simulink model "controlSpatialOrientation"  (R2025b)
settings: Solver=VariableStepAuto  StartTime=0.0  StopTime=100  RelTol=1e-3
undefined symbols (not defined in the file): C_T_pitch, C_T_rol, C_T_yaw, Ix, Iy, Iz
libraries: fuzblock x3
settings Model: Creator=torcik  LastModifiedBy=torcik

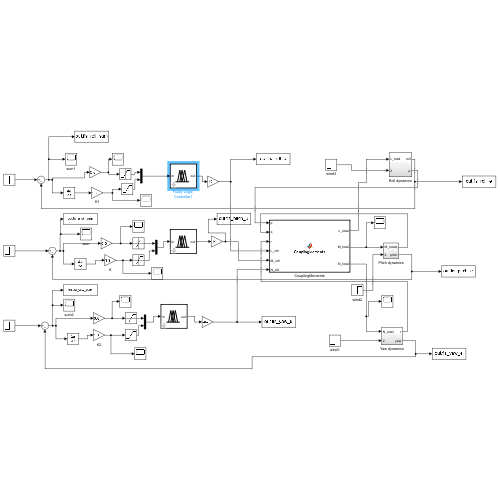
[thumbnail: Simulink's stored preview of the top-level diagram]
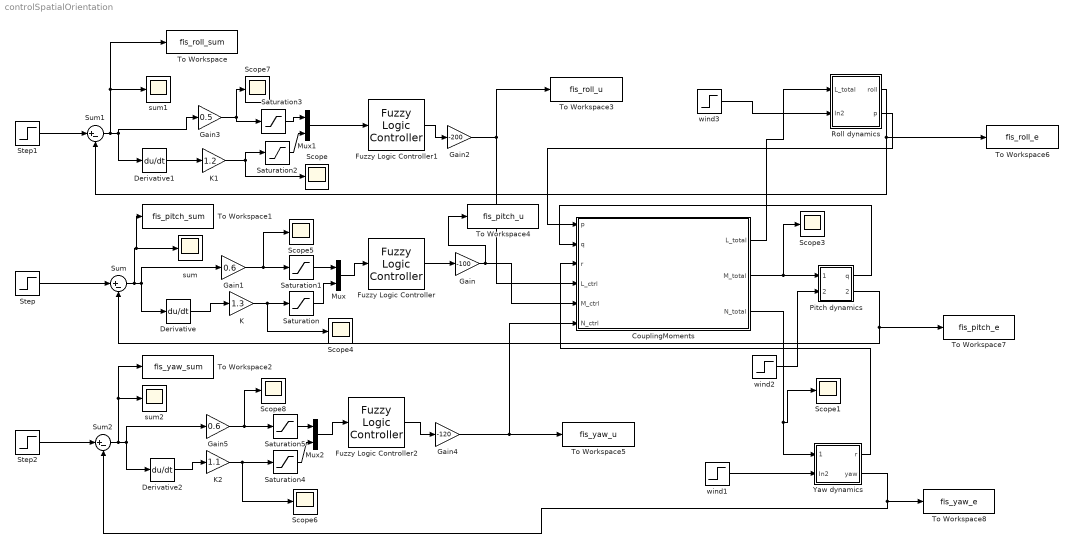
== system controlSpatialOrientation ==
  CouplingMoments : MATLAB Function  TreatAsAtomicUnit=on
  Derivative : Derivative
  Derivative1 : Derivative
  Derivative2 : Derivative
  Fuzzy Logic Controller : fuzblock/Fuzzy Logic  Controller  FIS='Mamdani_gauss'  OutputSampleNumber=101  DataType=double  UseLookupTable=off  NumBreakpoints=10  FuzzifiedInputs=off  RuleFiringStrengths=off  RuleOutputs=off  AggregatedOutputs=off  SimulateUsing=Interpreted execution  OutOfRangeInputValueMessage=warning  NoRuleFiredMessage=warning  EmptyOutputFuzzySetMessage=warning
  Fuzzy Logic Controller1 : fuzblock/Fuzzy Logic  Controller  FIS='Mamdani_gauss.fis'  OutputSampleNumber=101  DataType=double  UseLookupTable=off  NumBreakpoints=10  FuzzifiedInputs=off  RuleFiringStrengths=off  RuleOutputs=off  AggregatedOutputs=off  SimulateUsing=Interpreted execution  OutOfRangeInputValueMessage=warning  NoRuleFiredMessage=warning  EmptyOutputFuzzySetMessage=warning
  Fuzzy Logic Controller2 : fuzblock/Fuzzy Logic  Controller  FIS='Mamdani_gauss'  OutputSampleNumber=101  DataType=double  UseLookupTable=off  NumBreakpoints=10  FuzzifiedInputs=off  RuleFiringStrengths=off  RuleOutputs=off  AggregatedOutputs=off  SimulateUsing=Interpreted execution  OutOfRangeInputValueMessage=warning  NoRuleFiredMessage=warning  EmptyOutputFuzzySetMessage=warning
  Gain : Gain  Gain=-100
  Gain1 : Gain  Gain=0.6
  Gain2 : Gain  Gain=-200
  Gain3 : Gain  Gain=0.5
  Gain4 : Gain  Gain=-120
  Gain5 : Gain  Gain=0.6
  K : Gain  Gain=1.3
  K1 : Gain  Gain=1.2
  K2 : Gain  Gain=1.1
  Mux : Mux  Inputs=2
  Mux1 : Mux  Inputs=2
  Mux2 : Mux  Inputs=2
  Pitch dynamics : Subsystem
  Roll dynamics : Subsystem
  Saturation{,1..5} (6 alike) : Saturate  UpperLimit=1  LowerLimit=-1
  Scope{,1,3..8} (8 alike) : Scope
      Scope1 settings: ActiveDisplayYMinimum=-30.006205216170343  ActiveDisplayYMaximum=62.063006344123423
      Scope3 settings: ActiveDisplayYMinimum=-94.682244640541541  ActiveDisplayYMaximum=101.19826398937276  DataLoggingVariableName=ScopeData6
      Scope4 settings: ActiveDisplayYMinimum=-0.941753188542225  ActiveDisplayYMaximum=1.119037509535425  DataLoggingVariableName=ScopeData4
      Scope5 settings: ActiveDisplayYMinimum=-3.4905201219570272  ActiveDisplayYMaximum=4.8051428898956745  DataLoggingVariableName=ScopeData7
      Scope6 settings: ActiveDisplayYMinimum=-2.6378634590723506  ActiveDisplayYMaximum=2.3807373782151697  DataLoggingVariableName=ScopeData11
      Scope7 settings: ActiveDisplayYMinimum=-1.7145970677286446  ActiveDisplayYMaximum=2.8807785219943534  DataLoggingVariableName=ScopeData10
      Scope8 settings: ActiveDisplayYMinimum=-0.77533644485823927  ActiveDisplayYMaximum=0.60883418289029312  DataLoggingVariableName=ScopeData14
  Step : Step  After=0  SampleTime=0
  Step1 : Step  After=0  SampleTime=0
  Step2 : Step  After=0  SampleTime=0
  Sum : Sum  Inputs=|+-
  Sum1 : Sum  Inputs=|+-
  Sum2 : Sum  Inputs=|+-
  To Workspace : ToWorkspace  VariableName=fis_roll_sum  SaveFormat=Timeseries  SampleTime=-1
  To Workspace1 : ToWorkspace  VariableName=fis_pitch_sum  SaveFormat=Timeseries  SampleTime=-1
  To Workspace2 : ToWorkspace  VariableName=fis_yaw_sum  SaveFormat=Timeseries  SampleTime=-1
  To Workspace3 : ToWorkspace  VariableName=fis_roll_u  SaveFormat=Timeseries  SampleTime=-1
  To Workspace4 : ToWorkspace  VariableName=fis_pitch_u  SaveFormat=Timeseries  SampleTime=-1
  To Workspace5 : ToWorkspace  VariableName=fis_yaw_u  SaveFormat=Timeseries  SampleTime=-1
  To Workspace6 : ToWorkspace  VariableName=fis_roll_e  SaveFormat=Timeseries  SampleTime=-1
  To Workspace7 : ToWorkspace  VariableName=fis_pitch_e  SaveFormat=Timeseries  SampleTime=-1
  To Workspace8 : ToWorkspace  VariableName=fis_yaw_e  SaveFormat=Timeseries  SampleTime=-1
  Yaw dynamics : Subsystem
  sum : Scope
      settings: ActiveDisplayYMinimum=-11.524144518462831  ActiveDisplayYMaximum=17.172119250300984  DataLoggingVariableName=ScopeData3
  sum1 : Scope
      settings: ActiveDisplayYMinimum=-53.657968035336033  ActiveDisplayYMaximum=44.452232794535909  DataLoggingVariableName=ScopeData9
  sum2 : Scope
      settings: ActiveDisplayYMinimum=-20.980278823689279  ActiveDisplayYMaximum=22.797934110862389  DataLoggingVariableName=ScopeData13
  wind1 : Step  Time=10  After=5  SampleTime=0
  wind2 : Step  Time=10  After=5  SampleTime=0
  wind3 : Step  Time=10  After=5  SampleTime=0
  wires:
  Pitch dynamics/2(pitch) -> Sum/2, To Workspace7/1
  Step/1 -> Sum/1
  Derivative/1 -> K/1
  Mux/1 -> Fuzzy Logic Controller/1
  Sum/1 -> To Workspace1/1, sum/1, Derivative/1, Gain1/1
  K/1 -> Scope4/1, Saturation/1
  Saturation/1 -> Mux/2
  Gain1/1 -> Scope5/1, Saturation1/1
  Saturation1/1 -> Mux/1
  Roll dynamics/1(roll) -> To Workspace6/1, Sum1/2
  Mux1/1 -> Fuzzy Logic Controller1/1
  Saturation3/1 -> Mux1/1
  Fuzzy Logic Controller1/1 -> Gain2/1
  Derivative1/1 -> K1/1
  Sum1/1 -> sum1/1, To Workspace/1, Derivative1/1, Gain3/1
  Saturation2/1 -> Mux1/2
  Gain3/1 -> Scope7/1, Saturation3/1
  Step1/1 -> Sum1/1
  Yaw dynamics/2(yaw) -> To Workspace8/1, Sum2/2
  Mux2/1 -> Fuzzy Logic Controller2/1
  Saturation5/1 -> Mux2/1
  Derivative2/1 -> K2/1
  K2/1 -> Scope6/1, Saturation4/1
  Sum2/1 -> To Workspace2/1, sum2/1, Derivative2/1, Gain5/1
  Saturation4/1 -> Mux2/2
  Gain5/1 -> Scope8/1, Saturation5/1
  Step2/1 -> Sum2/1
  Fuzzy Logic Controller/1 -> Gain/1
  Fuzzy Logic Controller2/1 -> Gain4/1
  Gain4/1 -> CouplingMoments/6(N_ctrl), To Workspace5/1
  Gain/1 -> CouplingMoments/5(M_ctrl), To Workspace4/1
  Roll dynamics/2(p) -> CouplingMoments/1(p)
  Pitch dynamics/1(q) -> CouplingMoments/2(q)
  Yaw dynamics/1(r) -> CouplingMoments/3(r)
  Gain2/1 -> CouplingMoments/4(L_ctrl), To Workspace3/1
  CouplingMoments/1(L_total) -> Roll dynamics/1(L_total)
  CouplingMoments/2(M_total) -> Scope3/1, Pitch dynamics/1(M_total)
  CouplingMoments/3(N_total) -> Scope1/1, Yaw dynamics/1(N_total)
  K1/1 -> Scope/1, Saturation2/1
  wind1/1 -> Yaw dynamics/2(In2)
  wind2/1 -> Pitch dynamics/2(In2)
  wind3/1 -> Roll dynamics/2(In2)

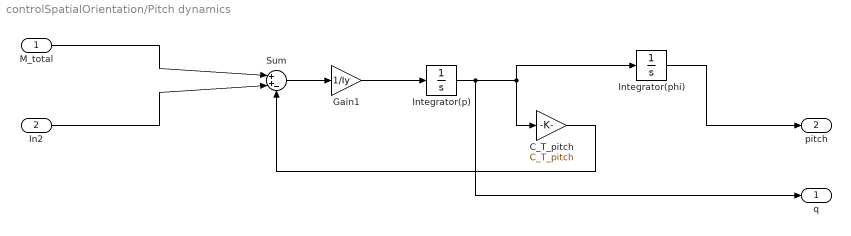
== system controlSpatialOrientation/Pitch dynamics ==
  M_total : Inport
  In2 : Inport  Port=2
  C_T_pitch : Gain  Gain=C_T_pitch
  Gain1 : Gain  Gain=1/Iy
  Integrator(p) : Integrator
  Integrator(phi) : Integrator
  Sum : Sum  Inputs=|++-
  q : Outport
  pitch : Outport  Port=2
  wires:
  Integrator(p)/1 -> q/1, Integrator(phi)/1, C_T_pitch/1
  C_T_pitch/1 -> Sum/3
  Integrator(phi)/1 -> pitch/1
  Gain1/1 -> Integrator(p)/1
  M_total/1 -> Sum/1
  Sum/1 -> Gain1/1
  In2/1 -> Sum/2

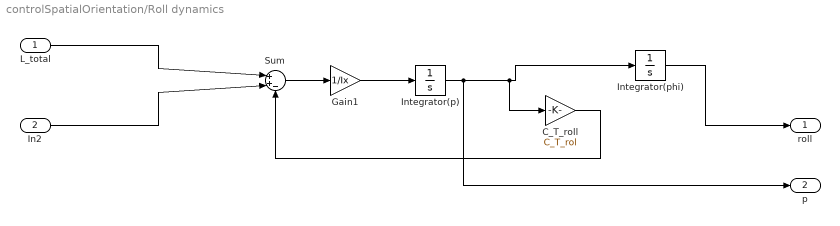
== system controlSpatialOrientation/Roll dynamics ==
  L_total : Inport
  In2 : Inport  Port=2
  C_T_roll : Gain  Gain=C_T_rol
  Gain1 : Gain  Gain=1/Ix
  Integrator(p) : Integrator
  Integrator(phi) : Integrator
  Sum : Sum  Inputs=|++-
  roll : Outport
  p : Outport  Port=2
  wires:
  Integrator(p)/1 -> p/1, Integrator(phi)/1, C_T_roll/1
  C_T_roll/1 -> Sum/3
  Integrator(phi)/1 -> roll/1
  Gain1/1 -> Integrator(p)/1
  L_total/1 -> Sum/1
  Sum/1 -> Gain1/1
  In2/1 -> Sum/2

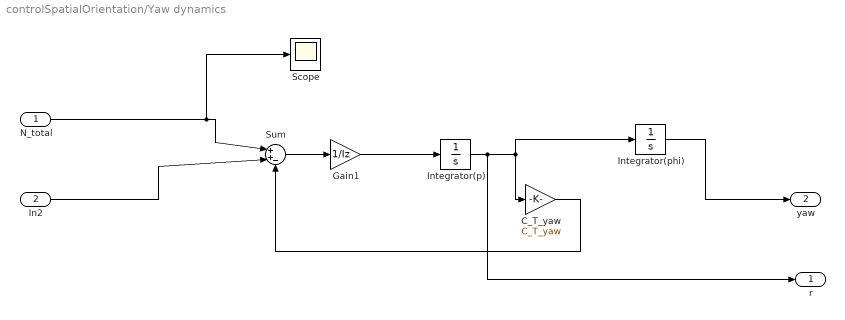
== system controlSpatialOrientation/Yaw dynamics ==
  N_total : Inport
  In2 : Inport  Port=2
  C_T_yaw : Gain  Gain=C_T_yaw
  Gain1 : Gain  Gain=1/Iz
  Integrator(p) : Integrator
  Integrator(phi) : Integrator
  Scope : Scope
      settings: ActiveDisplayYMinimum=-1  ActiveDisplayYMaximum=1  DataLoggingVariableName=ScopeData8
  Sum : Sum  Inputs=|++-
  r : Outport
  yaw : Outport  Port=2
  wires:
  Integrator(p)/1 -> r/1, Integrator(phi)/1, C_T_yaw/1
  C_T_yaw/1 -> Sum/3
  Integrator(phi)/1 -> yaw/1
  Gain1/1 -> Integrator(p)/1
  N_total/1 -> Scope/1, Sum/1
  Sum/1 -> Gain1/1
  In2/1 -> Sum/2

== matlab function controlSpatialOrientation/CouplingMoments ==
  data: p input; L_total output; q input; r input; L_ctrl input; M_ctrl input; N_ctrl input; M_total output; N_total output
function [L_total, M_total, N_total] = CouplingMoments(p, q, r, L_ctrl, M_ctrl, N_ctrl)


Ix = 100;     
Iy = 150;     
Iz = 200;  


L_coup = (Iy - Iz) * q * r;
M_coup = (Iz - Ix) * p * r;
N_coup = (Ix - Iy) * p * q;



L_total = L_ctrl + L_coup;
M_total = M_ctrl + M_coup;
N_total = N_ctrl + N_coup;
end
